simulink library "tramontina_database_sick_modbuslib"  (R2023b)
settings: Solver=VariableStepAuto  StartTime=0.0  StopTime=10.0  RelTol=1e-3
libraries: canmsglib x4, simulink x1
settings Model: Creator=matlab.cut  LastModifiedBy=matlab.cut

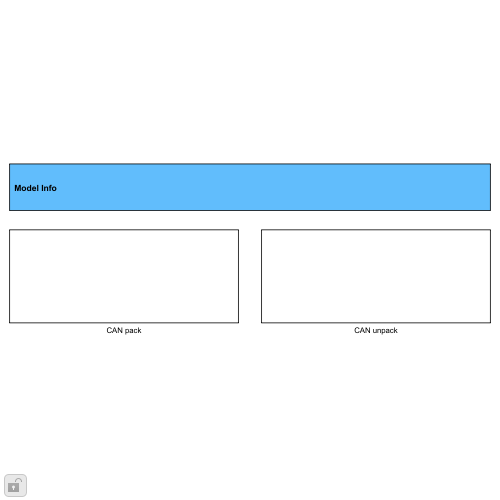
[thumbnail: Simulink's stored preview of the top-level diagram]
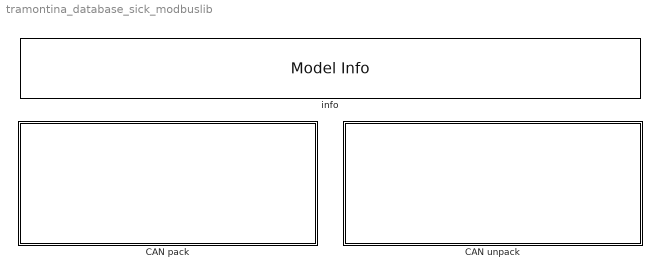
== system tramontina_database_sick_modbuslib ==
  CAN pack : Subsystem
  CAN unpack : Subsystem
  info : simulink/Model-Wide Utilities/Model Info  Frame=on  DisplayStringWithTags=SPEEDGOAT CAN Database Library for: tramontina_database_sick_modbus  HorizontalTextAlignment=Left  LeftAlignmentValue=0.01

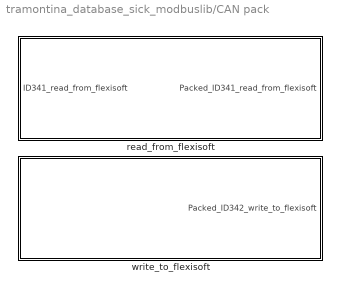
== system tramontina_database_sick_modbuslib/CAN pack ==
  read_from_flexisoft : Subsystem
  write_to_flexisoft : Subsystem

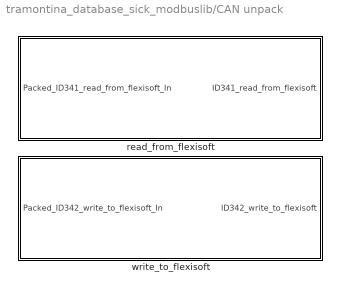
== system tramontina_database_sick_modbuslib/CAN unpack ==
  read_from_flexisoft : Subsystem
  write_to_flexisoft : Subsystem

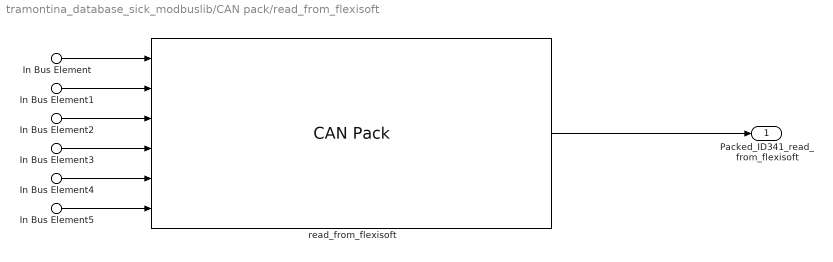
== system tramontina_database_sick_modbuslib/CAN pack/read_from_flexisoft ==
  In Bus Element : Inport  PortName=ID341_read_from_flexisoft  Element=AuxEmEmergencia
  In Bus Element1 : Inport  PortName=ID341_read_from_flexisoft  Element=AuxScannerInterrompido
  In Bus Element2 : Inport  PortName=ID341_read_from_flexisoft  Element=EmergenciaFrontalDireita
  In Bus Element3 : Inport  PortName=ID341_read_from_flexisoft  Element=EmergenciaFrontalEsquerda
  In Bus Element4 : Inport  PortName=ID341_read_from_flexisoft  Element=EmergenciaTraseiraDireita
  In Bus Element5 : Inport  PortName=ID341_read_from_flexisoft  Element=EmergenciaTraseiraEsquerda
  read_from_flexisoft : canmsglib/CAN Pack  CANdbFile=C:\Users\matlab.cut\Desktop\AMR\canbus_files\tramontina_database_sick_modbus.dbc  MsgList=read_from_flexisoft  MsgName=read_from_flexisoft  MsgIDType=Standard (11-bit identifier)  MsgIdentifier=341  MsgLength=4  Remote=off  ApplyMinMax=off  BusOutput=on  SignalInfo={'AuxEmEmergencia','0','1','LE','unsigned','Standard','0','1','0','0','1';'AuxScannerInterrompido','1','1','LE','unsigned','Standard','0','1','0','0','1';'EmergenciaFrontalDireita','16','1','LE','unsigned','Standard','0','1','0','0','1';'EmergenciaFrontalEsquerda','18','1','LE','unsigned','Standard','0','1','0','0','1';'EmergenciaTraseiraDireita','20','1','LE','unsigned','Standard','0','1','0','0','1';'EmergenciaTraseiraEsquerda','22','1','LE','unsigned','Standard','0','1','0','0','1'}
      settings: DataFormat=manually specified signals
  Packed_ID341_read_from_flexisoft : Outport
  wires:
  read_from_flexisoft/1 -> Packed_ID341_read_from_flexisoft/1
  In Bus Element/1 -> read_from_flexisoft/1
  In Bus Element1/1 -> read_from_flexisoft/2
  In Bus Element2/1 -> read_from_flexisoft/3
  In Bus Element3/1 -> read_from_flexisoft/4
  In Bus Element4/1 -> read_from_flexisoft/5
  In Bus Element5/1 -> read_from_flexisoft/6

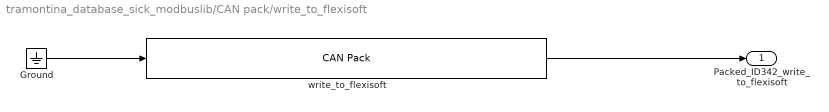
== system tramontina_database_sick_modbuslib/CAN pack/write_to_flexisoft ==
  Ground : Ground
  write_to_flexisoft : canmsglib/CAN Pack  CANdbFile=C:\Users\matlab.cut\Desktop\AMR\canbus_files\tramontina_database_sick_modbus.dbc  MsgList=write_to_flexisoft  MsgName=write_to_flexisoft  MsgIDType=Standard (11-bit identifier)  MsgIdentifier=342  MsgLength=4  Remote=off  ApplyMinMax=off  BusOutput=on  SignalInfo={}
      settings: DataFormat=manually specified signals
  Packed_ID342_write_to_flexisoft : Outport
  wires:
  write_to_flexisoft/1 -> Packed_ID342_write_to_flexisoft/1
  Ground/1 -> write_to_flexisoft/1

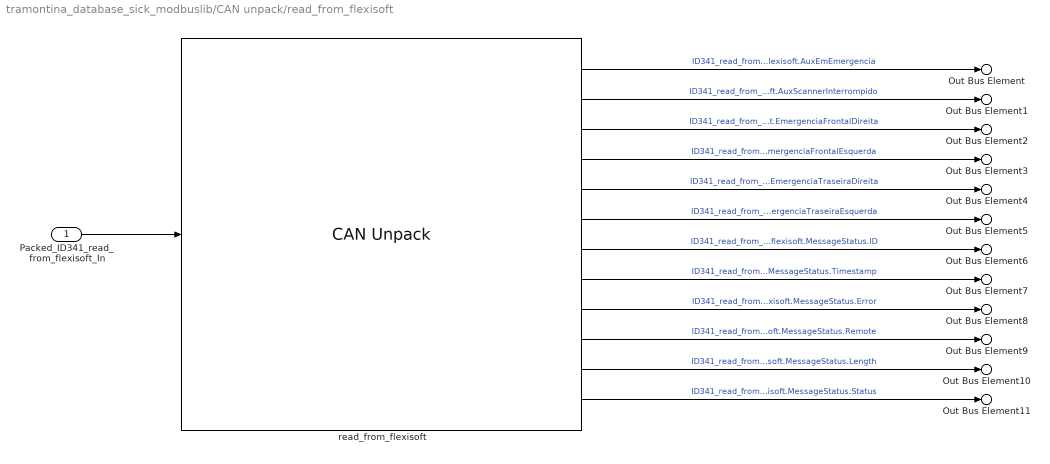
== system tramontina_database_sick_modbuslib/CAN unpack/read_from_flexisoft ==
  Packed_ID341_read_from_flexisoft_In : Inport
  read_from_flexisoft : canmsglib/CAN Unpack  CANdbFile=C:\Users\matlab.cut\Desktop\AMR\canbus_files\tramontina_database_sick_modbus.dbc  MsgList=read_from_flexisoft  MsgName=read_from_flexisoft  MsgIDType=Standard (11-bit identifier)  MsgIdentifier=341  MsgLength=4  SignalInfo={'AuxEmEmergencia','0','1','LE','unsigned','Standard','0','1','0','0','1';'AuxScannerInterrompido','1','1','LE','unsigned','Standard','0','1','0','0','1';'EmergenciaFrontalDireita','16','1','LE','unsigned','Standard','0','1','0','0','1';'EmergenciaFrontalEsquerda','18','1','LE','unsigned','Standard','0','1','0','0','1';'EmergenciaTraseiraDireita','20','1','LE','unsigned','Standard','0','1','0','0','1';'EmergenciaTraseiraEsquerda','22','1','LE','unsigned','Standard','0','1','0','0','1'}  IDPort=on  TimestampPort=on  ErrorPort=on  RemotePort=on  LengthPort=on  StatusPort=on  ApplyMinMax=off
  Out Bus Element : Outport  PortName=ID341_read_from_flexisoft  Element=AuxEmEmergencia
  Out Bus Element1 : Outport  PortName=ID341_read_from_flexisoft  Element=AuxScannerInterrompido
  Out Bus Element2 : Outport  PortName=ID341_read_from_flexisoft  Element=EmergenciaFrontalDireita
  Out Bus Element3 : Outport  PortName=ID341_read_from_flexisoft  Element=EmergenciaFrontalEsquerda
  Out Bus Element4 : Outport  PortName=ID341_read_from_flexisoft  Element=EmergenciaTraseiraDireita
  Out Bus Element5 : Outport  PortName=ID341_read_from_flexisoft  Element=EmergenciaTraseiraEsquerda
  Out Bus Element6 : Outport  PortName=ID341_read_from_flexisoft  Element=MessageStatus.ID
  Out Bus Element7 : Outport  PortName=ID341_read_from_flexisoft  Element=MessageStatus.Timestamp
  Out Bus Element8 : Outport  PortName=ID341_read_from_flexisoft  Element=MessageStatus.Error
  Out Bus Element9 : Outport  PortName=ID341_read_from_flexisoft  Element=MessageStatus.Remote
  Out Bus Element10 : Outport  PortName=ID341_read_from_flexisoft  Element=MessageStatus.Length
  Out Bus Element11 : Outport  PortName=ID341_read_from_flexisoft  Element=MessageStatus.Status
  wires:
  Packed_ID341_read_from_flexisoft_In/1 -> read_from_flexisoft/1
  read_from_flexisoft/1 -> Out Bus Element/1  "ID341_read_from_flexisoft.AuxEmEmergencia"
  read_from_flexisoft/2 -> Out Bus Element1/1  "ID341_read_from_flexisoft.AuxScannerInterrompido"
  read_from_flexisoft/3 -> Out Bus Element2/1  "ID341_read_from_flexisoft.EmergenciaFrontalDireita"
  read_from_flexisoft/4 -> Out Bus Element3/1  "ID341_read_from_flexisoft.EmergenciaFrontalEsquerda"
  read_from_flexisoft/5 -> Out Bus Element4/1  "ID341_read_from_flexisoft.EmergenciaTraseiraDireita"
  read_from_flexisoft/6 -> Out Bus Element5/1  "ID341_read_from_flexisoft.EmergenciaTraseiraEsquerda"
  read_from_flexisoft/7 -> Out Bus Element6/1  "ID341_read_from_flexisoft.MessageStatus.ID"
  read_from_flexisoft/8 -> Out Bus Element7/1  "ID341_read_from_flexisoft.MessageStatus.Timestamp"
  read_from_flexisoft/9 -> Out Bus Element8/1  "ID341_read_from_flexisoft.MessageStatus.Error"
  read_from_flexisoft/10 -> Out Bus Element9/1  "ID341_read_from_flexisoft.MessageStatus.Remote"
  read_from_flexisoft/11 -> Out Bus Element10/1  "ID341_read_from_flexisoft.MessageStatus.Length"
  read_from_flexisoft/12 -> Out Bus Element11/1  "ID341_read_from_flexisoft.MessageStatus.Status"

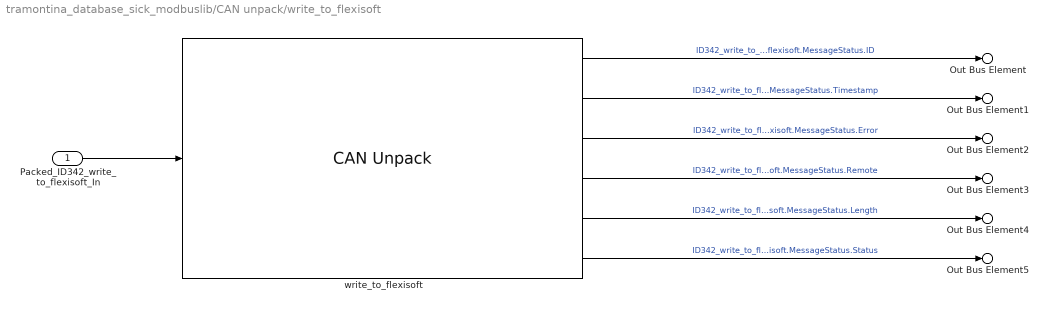
== system tramontina_database_sick_modbuslib/CAN unpack/write_to_flexisoft ==
  Packed_ID342_write_to_flexisoft_In : Inport
  write_to_flexisoft : canmsglib/CAN Unpack  CANdbFile=C:\Users\matlab.cut\Desktop\AMR\canbus_files\tramontina_database_sick_modbus.dbc  MsgList=write_to_flexisoft  MsgName=write_to_flexisoft  MsgIDType=Standard (11-bit identifier)  MsgIdentifier=342  MsgLength=4  SignalInfo={}  IDPort=on  TimestampPort=on  ErrorPort=on  RemotePort=on  LengthPort=on  StatusPort=on  ApplyMinMax=off
  Out Bus Element : Outport  PortName=ID342_write_to_flexisoft  Element=MessageStatus.ID
  Out Bus Element1 : Outport  PortName=ID342_write_to_flexisoft  Element=MessageStatus.Timestamp
  Out Bus Element2 : Outport  PortName=ID342_write_to_flexisoft  Element=MessageStatus.Error
  Out Bus Element3 : Outport  PortName=ID342_write_to_flexisoft  Element=MessageStatus.Remote
  Out Bus Element4 : Outport  PortName=ID342_write_to_flexisoft  Element=MessageStatus.Length
  Out Bus Element5 : Outport  PortName=ID342_write_to_flexisoft  Element=MessageStatus.Status
  wires:
  Packed_ID342_write_to_flexisoft_In/1 -> write_to_flexisoft/1
  write_to_flexisoft/1 -> Out Bus Element/1  "ID342_write_to_flexisoft.MessageStatus.ID"
  write_to_flexisoft/2 -> Out Bus Element1/1  "ID342_write_to_flexisoft.MessageStatus.Timestamp"
  write_to_flexisoft/3 -> Out Bus Element2/1  "ID342_write_to_flexisoft.MessageStatus.Error"
  write_to_flexisoft/4 -> Out Bus Element3/1  "ID342_write_to_flexisoft.MessageStatus.Remote"
  write_to_flexisoft/5 -> Out Bus Element4/1  "ID342_write_to_flexisoft.MessageStatus.Length"
  write_to_flexisoft/6 -> Out Bus Element5/1  "ID342_write_to_flexisoft.MessageStatus.Status"
